simulink model "funRamp"  (Simulink 7.9)
settings: Solver=ode45  StartTime=0.0  StopTime=5  RelTol=1e-9
libraries: simulink x1
settings Model: Creator=ex16  LastModifiedBy=ex16

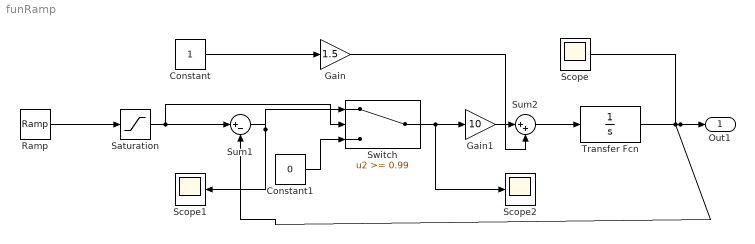
== system funRamp ==
  Constant : Constant
  Constant1 : Constant  Value=0
  Gain : Gain  Gain=1.5
  Gain1 : Gain  Gain=10
  Ramp : simulink/Sources/Ramp  slope=1  start=0  X0=0
  Saturation : Saturate  UpperLimit=1  LowerLimit=0
  Scope : Scope
  Scope1 : Scope
  Scope2 : Scope
      settings: SaveName=ScopeData2
  Sum1 : Sum  Inputs=|+-
  Sum2 : Sum  Inputs=|++
  Switch : Switch  Threshold=0.99
  Transfer Fcn : TransferFcn  Denominator=[1 0]
  Out1 : Outport
  wires:
  Transfer Fcn/1 -> Out1/1, Scope/1, Sum1/2
  Sum2/1 -> Transfer Fcn/1
  Gain/1 -> Sum2/2
  Saturation/1 -> Sum1/1, Switch/2
  Ramp/1 -> Saturation/1
  Gain1/1 -> Sum2/1
  Sum1/1 -> Scope1/1, Switch/1
  Constant/1 -> Gain/1
  Switch/1 -> Gain1/1, Scope2/1
  Constant1/1 -> Switch/3
